simulink model "tempJump_"  (R2015b)
settings: Solver=FixedStepDiscrete  StartTime=0.0  StopTime=1.0  FixedStep=1.0  RelTol=1e-3
libraries: taXlibrary x5
settings Model: Creator=emmert  LastModifiedBy=thomas
settings DataIOCC: SaveFormat=Array  SignalLoggingSaveFormat=ModelDataLogs
settings OptimizationCC: ExpressionDepthLimit=2147483647
settings DebuggingCC: UnderspecifiedInitializationDetection=Classic  MergeDetectMultiDrivingBlocksExec=none  SolverPrmCheckMsg=warning  FcnCallInpInsideContextMsg=EnableAllAsWarning  StateNameClashWarn=warning
settings HardwareCC: ProdBitPerPointer=32  ProdLargestAtomicFloat=None  ProdIntDivRoundTo=Undefined  ProdEndianess=Unspecified  ProdWordSize=32  ProdHWDeviceType=32-bit Generic
settings GRTTargetCC: GeneratePreprocessorConditionals=Disable all  CombineOutputUpdateFcns=off  GRTInterface=on
settings ConfigComp: CovModelRefEnable=Off

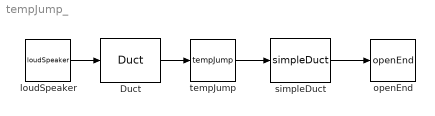
== system tempJump_ ==
  Duct : taXlibrary/Duct  element=Duct  order=3  minres=40  l=0.5  sensorPositions=[]
      settings: AttributesFormatString=%<l> m
  loudSpeaker : taXlibrary/loudSpeaker  element=loudSpeaker  loc=Upstream  Amp=1  A=1.4  Mach=0.1  rho=1.2  c=100
      settings: AttributesFormatString=%<Amp> m/s
  openEnd : taXlibrary/openEnd  element=openEnd  loc=Downstream  A=[]  Mach=[]  rho=[]  c=[]
  simpleDuct : taXlibrary/simpleDuct  element=simpleDuct  l=0.25  damping_model_popup=no damping  gm=1.4  nu=1.568e-5  Pr=5  damping_model_id=1
      settings: AttributesFormatString=%<l> m
  tempJump : taXlibrary/tempJump  element=tempJump  Mach=0.3  rho=0.29  c=287
  wires:
  loudSpeaker/1 -> Duct/1
  simpleDuct/1 -> openEnd/1
  Duct/1 -> tempJump/1
  tempJump/1 -> simpleDuct/1
